simulink model "test_COM"  (Simulink 8.7)
settings: Solver=ode45  StartTime=0.0  StopTime=2  MaxStep=Step_Time  RelTol=1e-3
settings Model: Creator=saeed  LastModifiedBy=Other
settings DataIOCC: SignalLoggingSaveFormat=ModelDataLogs
settings OptimizationCC: ExpressionDepthLimit=2147483647
settings DebuggingCC: SolverPrmCheckMsg=warning  FcnCallInpInsideContextMsg=UseLocalSettings  StateNameClashWarn=warning
settings GRTTargetCC: CombineOutputUpdateFcns=off  GRTInterface=on

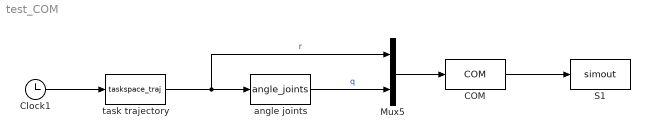
== system test_COM ==
  COM : MATLABFcn  MATLABFcn=COM
  Clock1 : Clock
  Mux5 : Mux  Inputs=2
  S1 : ToWorkspace  VariableName=simout  SaveFormat=Structure With Time  SampleTime=-1
  angle joints : MATLABFcn  MATLABFcn=angle_joints
  task trajectory : MATLABFcn  MATLABFcn=taskspace_traj
  wires:
  Clock1/1 -> task trajectory/1
  task trajectory/1 -> Mux5/1, angle joints/1  "r"
  COM/1 -> S1/1
  Mux5/1 -> COM/1
  angle joints/1 -> Mux5/2  "q"
